simulink model "CyberDog_Motor_FOC_preRefactor_20260807_213408"  (R2025b)
settings: Solver=FixedStepDiscrete  StartTime=0.0  StopTime=0.5  FixedStep=0.0001  RelTol=1e-3
InitFcn:
  | p = fileparts(get_param(bdroot,'FileName')); addpath(fullfile(p,'scripts')); motor_params;
undefined symbols (not defined in the file): Cogging_Lut_Angle, Cogging_Lut_V, CoggingFF_En, Curr_MaxOut, Curr_MinOut, CurrD_Ki, CurrD_Kp, CurrQ_Ki, CurrQ_Kp, DeadComp_En, DeadComp_Lut_I, DeadComp_Lut_V, DiscIntNeverNeededParam, MaxMod, Speed_Ki, Speed_Kp, Speed_Loop_N, Speed_MaxOut, Speed_MinOut, Vbus_nom
settings Model: Creator=Baseline  LastModifiedBy=Baseline

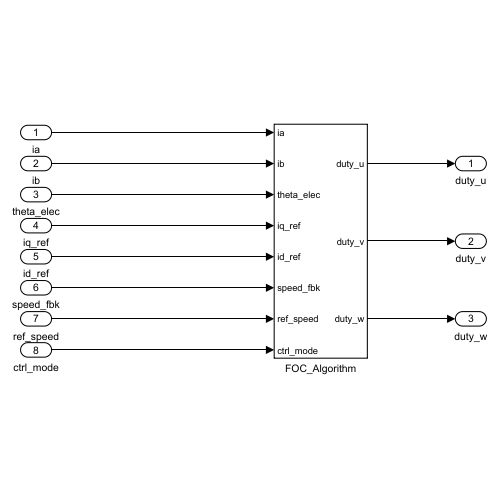
[thumbnail: Simulink's stored preview of the top-level diagram]
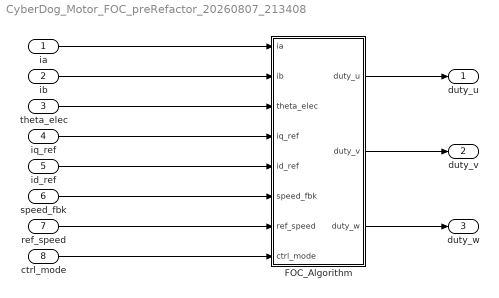
== system CyberDog_Motor_FOC_preRefactor_20260807_213408 ==
  ia : Inport
  ib : Inport  Port=2
  theta_elec : Inport  Port=3
  iq_ref : Inport  Port=4
  id_ref : Inport  Port=5
  speed_fbk : Inport  Port=6
  ref_speed : Inport  Port=7
  ctrl_mode : Inport  Port=8
  FOC_Algorithm : Subsystem
  duty_u : Outport
  duty_v : Outport  Port=2
  duty_w : Outport  Port=3
  wires:
  ctrl_mode/1 -> FOC_Algorithm/8(ctrl_mode)
  ref_speed/1 -> FOC_Algorithm/7(ref_speed)
  speed_fbk/1 -> FOC_Algorithm/6(speed_fbk)
  ia/1 -> FOC_Algorithm/1(ia)
  ib/1 -> FOC_Algorithm/2(ib)
  theta_elec/1 -> FOC_Algorithm/3(theta_elec)
  iq_ref/1 -> FOC_Algorithm/4(iq_ref)
  id_ref/1 -> FOC_Algorithm/5(id_ref)
  FOC_Algorithm/1(duty_u) -> duty_u/1
  FOC_Algorithm/2(duty_v) -> duty_v/1
  FOC_Algorithm/3(duty_w) -> duty_w/1

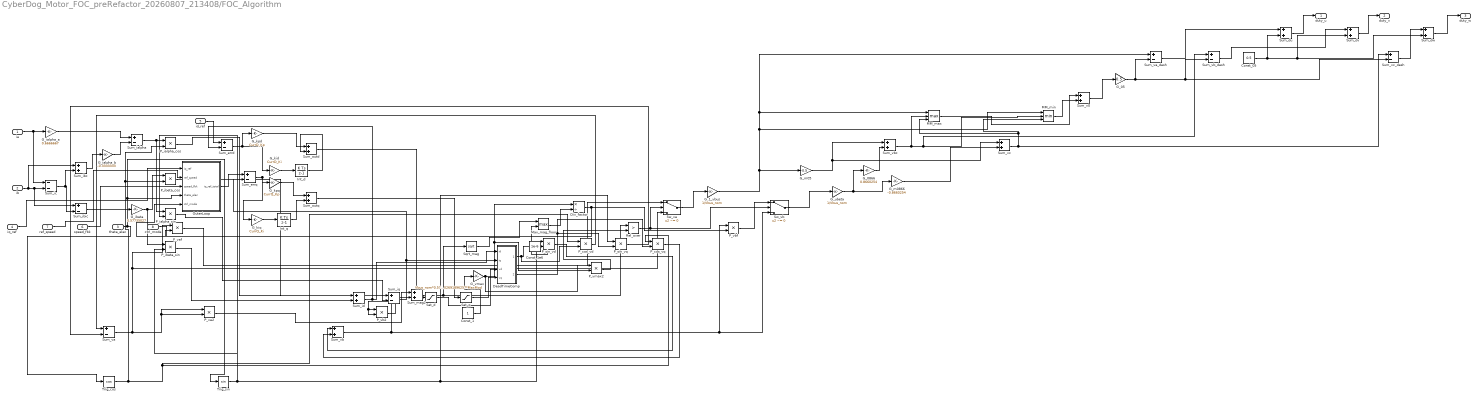
== system CyberDog_Motor_FOC_preRefactor_20260807_213408/FOC_Algorithm ==
  ia : Inport
  ib : Inport  Port=2
  theta_elec : Inport  Port=3
  iq_ref : Inport  Port=4
  id_ref : Inport  Port=5
  speed_fbk : Inport  Port=6
  ref_speed : Inport  Port=7
  ctrl_mode : Inport  Port=8
  Const_05 : Constant  Value=0.5
  Const_1 : Constant
  Const_1e6 : Constant  Value=1e-6
  DeadTimeComp : Subsystem
  Div_factor : Product  Inputs=*/
  G_05 : Gain  Gain=0.5
  G_0866 : Gain  Gain=0.8660254
  G_1_vbus : Gain  Gain=1/Vbus_nom
  G_ialpha_a : Gain  Gain=0.6666667
  G_ialpha_b : Gain  Gain=-0.3333333
  G_ibeta : Gain  Gain=0.57735027
  G_kid : Gain  Gain=CurrD_Ki
  G_kiq : Gain  Gain=CurrQ_Ki
  G_kpd : Gain  Gain=CurrD_Kp
  G_kpq : Gain  Gain=CurrQ_Kp
  G_m05 : Gain  Gain=-0.5
  G_m0866 : Gain  Gain=-0.8660254
  G_ubeta : Gain  Gain=1/Vbus_nom
  G_vmax : Gain  Gain=Vbus_nom*0.5773502691896257*MaxMod
  Int_d : DiscreteIntegrator  SampleTime=-1  LimitOutput=on  UpperSaturationLimit=Curr_MaxOut  LowerSaturationLimit=Curr_MinOut  ICPrevOutput=DiscIntNeverNeededParam  ICPrevScaledInput=DiscIntNeverNeededParam
  Int_q : DiscreteIntegrator  SampleTime=-1  LimitOutput=on  UpperSaturationLimit=Curr_MaxOut  LowerSaturationLimit=Curr_MinOut  ICPrevOutput=DiscIntNeverNeededParam  ICPrevScaledInput=DiscIntNeverNeededParam
  MM_max : MinMax  Function=max  Inputs=3
  MM_min : MinMax  Inputs=3
  Max_mag_floor : MinMax  Function=max  Inputs=2
  OuterLoop : Subsystem
  P_cos_vd : Product  Inputs=**
  P_cos_vq : Product  Inputs=**
  P_ialpha_cos : Product  Inputs=**
  P_ialpha_sin : Product  Inputs=**
  P_ibeta_cos : Product  Inputs=**
  P_ibeta_sin : Product  Inputs=**
  P_sin_vd : Product  Inputs=**
  P_sin_vq : Product  Inputs=**
  P_va2 : Product  Inputs=**
  P_vaf : Product  Inputs=**
  P_vb2 : Product  Inputs=**
  P_vbf : Product  Inputs=**
  P_vmax2 : Product  Inputs=**
  Rel_over : RelationalOperator  Operator=>  OutDataTypeStr=boolean  RndMeth=Simplest  InputSameDT=off
  Sat_d : Saturate  UpperLimit=Curr_MaxOut  LowerLimit=Curr_MinOut
  Sat_q : Saturate  UpperLimit=Curr_MaxOut  LowerLimit=Curr_MinOut
  Sqrt_mag : Sqrt
  Sum_du : Sum
  Sum_dv : Sum
  Sum_dw : Sum
  Sum_errd : Sum  Inputs=+-
  Sum_errq : Sum  Inputs=+-
  Sum_ialpha : Sum  Inputs=+-
  Sum_ibc : Sum
  Sum_ibic : Sum  Inputs=+-
  Sum_ic : Sum  Inputs=--
  Sum_id : Sum
  Sum_iq : Sum  Inputs=+-
  Sum_mag2 : Sum
  Sum_outd : Sum
  Sum_outq : Sum
  Sum_v0 : Sum
  Sum_va : Sum  Inputs=+-
  Sum_va_dash : Sum  Inputs=+-
  Sum_vb : Sum
  Sum_vb_dash : Sum  Inputs=+-
  Sum_vbc : Sum
  Sum_vc : Sum
  Sum_vc_dash : Sum  Inputs=+-
  Sw_va : Switch  Criteria=u2 ~= 0  SaturateOnIntegerOverflow=off  InputSameDT=off
  Sw_vb : Switch  Criteria=u2 ~= 0  SaturateOnIntegerOverflow=off  InputSameDT=off
  Trig_cos : Trigonometry  Operator=cos
  Trig_sin : Trigonometry
  duty_u : Outport
  duty_v : Outport  Port=2
  duty_w : Outport  Port=3
  wires:
  G_kpd/1 -> Sum_outd/1
  id_ref/1 -> Sum_errd/1
  Int_q/1 -> Sum_outq/2
  G_kiq/1 -> Int_q/1
  G_ibeta/1 -> P_ibeta_cos/1, P_ibeta_sin/1
  Sum_ialpha/1 -> P_ialpha_sin/1, P_ialpha_cos/1
  Sum_ibic/1 -> G_ibeta/1
  G_ialpha_b/1 -> Sum_ialpha/2
  G_ialpha_a/1 -> Sum_ialpha/1
  Sum_ibc/1 -> G_ialpha_b/1
  Sum_ic/1 -> Sum_ibic/2, Sum_ibc/2
  ib/1 -> Sum_ibic/1, Sum_ic/2, Sum_ibc/1
  ia/1 -> G_ialpha_a/1, Sum_ic/1
  Sum_dw/1 -> duty_w/1
  Sum_dv/1 -> duty_v/1
  Sum_du/1 -> duty_u/1
  Sum_vc_dash/1 -> Sum_dw/1
  Sum_vb_dash/1 -> Sum_dv/1
  Const_05/1 -> Sum_dw/2, Sum_dv/2, Sum_du/2
  Sum_va_dash/1 -> Sum_du/1
  G_05/1 -> Sum_vc_dash/2, Sum_vb_dash/2, Sum_va_dash/2
  Sum_v0/1 -> G_05/1
  MM_min/1 -> Sum_v0/2
  MM_max/1 -> Sum_v0/1
  Sum_vc/1 -> MM_min/3, MM_max/3, Sum_vc_dash/1
  Sum_vbc/1 -> Sum_vb_dash/1, MM_min/2, MM_max/2
  G_m0866/1 -> Sum_vc/2
  G_0866/1 -> Sum_vbc/2
  G_m05/1 -> Sum_vc/1, Sum_vbc/1
  G_ubeta/1 -> G_m0866/1, G_0866/1
  G_1_vbus/1 -> Sum_va_dash/1, MM_max/1, MM_min/1, G_m05/1
  Sw_vb/1 -> G_ubeta/1
  Sw_va/1 -> G_1_vbus/1
  P_vbf/1 -> Sw_vb/1
  Rel_over/1 -> Sw_vb/2, Sw_va/2
  P_vb2/1 -> Sum_mag2/2
  P_va2/1 -> Sum_mag2/1
  Sum_vb/1 -> Sw_vb/3, P_vbf/1, P_vb2/2, P_vb2/1
  Max_mag_floor/1 -> Div_factor/2
  Sum_mag2/1 -> Rel_over/1, Sqrt_mag/1
  Sqrt_mag/1 -> Max_mag_floor/1
  OuterLoop/1(iq_ref_total) -> Sum_errq/1
  ctrl_mode/1 -> OuterLoop/5(ctrl_mode)
  speed_fbk/1 -> OuterLoop/3(speed_fbk)
  ref_speed/1 -> OuterLoop/2(ref_speed)
  Div_factor/1 -> P_vbf/2, P_vaf/2
  theta_elec/1 -> OuterLoop/4(theta_elec), Trig_sin/1, Trig_cos/1
  Sum_va/1 -> P_va2/1, P_va2/2, P_vaf/1, Sw_va/3
  P_vaf/1 -> Sw_va/1
  iq_ref/1 -> OuterLoop/1(iq_ref)
  Sum_errq/1 -> G_kpq/1, G_kiq/1
  G_kpq/1 -> Sum_outq/1
  Sum_errd/1 -> G_kpd/1, G_kid/1
  G_kid/1 -> Int_d/1
  Int_d/1 -> Sum_outd/2
  DeadTimeComp/2(vq_out) -> P_cos_vq/2, P_sin_vq/2
  DeadTimeComp/1(vd_out) -> P_sin_vd/2, P_cos_vd/2
  Sum_iq/1 -> DeadTimeComp/2(iq), Sum_errq/2
  P_ialpha_sin/1 -> Sum_iq/2
  P_ibeta_cos/1 -> Sum_iq/1
  G_vmax/1 -> P_vmax2/2, Div_factor/1, P_vmax2/1
  Const_1e6/1 -> Max_mag_floor/2
  Sum_outd/1 -> Sat_d/1
  Sum_outq/1 -> Sat_q/1
  Trig_sin/1 -> P_sin_vq/1, P_sin_vd/1, P_ialpha_sin/2, P_ibeta_sin/2
  Trig_cos/1 -> P_cos_vd/1, P_cos_vq/1, P_ibeta_cos/2, P_ialpha_cos/2
  Sat_d/1 -> DeadTimeComp/3(vd)
  Sat_q/1 -> DeadTimeComp/4(vq)
  P_cos_vd/1 -> Sum_va/1
  P_sin_vq/1 -> Sum_va/2
  P_sin_vd/1 -> Sum_vb/1
  P_cos_vq/1 -> Sum_vb/2
  Const_1/1 -> G_vmax/1
  P_vmax2/1 -> Rel_over/2
  P_ialpha_cos/1 -> Sum_id/1
  P_ibeta_sin/1 -> Sum_id/2
  Sum_id/1 -> DeadTimeComp/1(id), Sum_errd/2

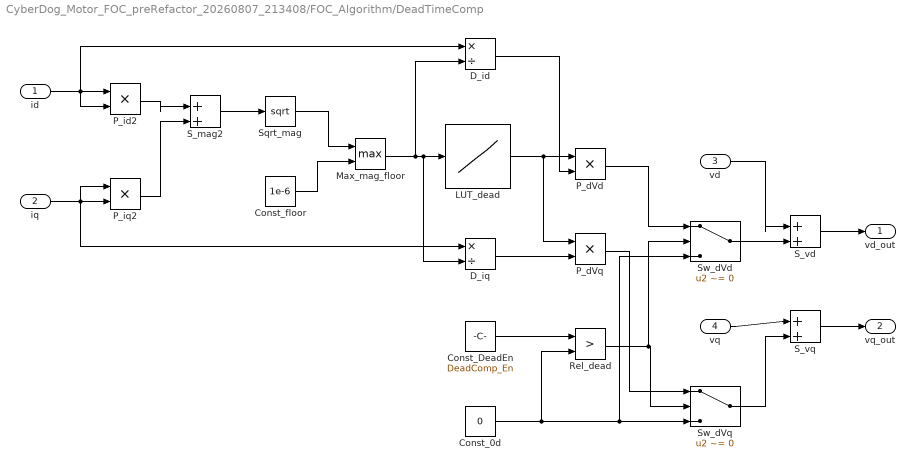
== system CyberDog_Motor_FOC_preRefactor_20260807_213408/FOC_Algorithm/DeadTimeComp ==
  id : Inport
  iq : Inport  Port=2
  vd : Inport  Port=3
  vq : Inport  Port=4
  Const_0d : Constant  Value=0
  Const_DeadEn : Constant  Value=DeadComp_En
  Const_floor : Constant  Value=1e-6
  D_id : Product  Inputs=*/
  D_iq : Product  Inputs=*/
  LUT_dead : Lookup_n-D  NumberOfTableDimensions=1  BreakpointsForDimension1=DeadComp_Lut_I  Table=DeadComp_Lut_V  InternalRulePriority=Speed  RndMeth=Simplest
  Max_mag_floor : MinMax  Function=max  Inputs=2
  P_dVd : Product  Inputs=**
  P_dVq : Product  Inputs=**
  P_id2 : Product  Inputs=**
  P_iq2 : Product  Inputs=**
  Rel_dead : RelationalOperator  Operator=>  OutDataTypeStr=boolean  RndMeth=Simplest  InputSameDT=off
  S_mag2 : Sum  Inputs=|++
  S_vd : Sum  Inputs=|++
  S_vq : Sum  Inputs=|++
  Sqrt_mag : Sqrt
  Sw_dVd : Switch  Criteria=u2 ~= 0  SaturateOnIntegerOverflow=off  InputSameDT=off
  Sw_dVq : Switch  Criteria=u2 ~= 0  SaturateOnIntegerOverflow=off  InputSameDT=off
  vd_out : Outport
  vq_out : Outport  Port=2
  wires:
  S_vq/1 -> vq_out/1
  S_vd/1 -> vd_out/1
  Sw_dVq/1 -> S_vq/2
  vq/1 -> S_vq/1
  Sw_dVd/1 -> S_vd/2
  vd/1 -> S_vd/1
  Const_DeadEn/1 -> Rel_dead/1
  P_dVq/1 -> Sw_dVq/1
  Const_0d/1 -> Sw_dVd/3, Sw_dVq/3, Rel_dead/2
  Rel_dead/1 -> Sw_dVd/2, Sw_dVq/2
  P_dVd/1 -> Sw_dVd/1
  D_iq/1 -> P_dVq/2
  D_id/1 -> P_dVd/2
  LUT_dead/1 -> P_dVd/1, P_dVq/1
  Max_mag_floor/1 -> LUT_dead/1, D_iq/2, D_id/2
  Const_floor/1 -> Max_mag_floor/2
  Sqrt_mag/1 -> Max_mag_floor/1
  S_mag2/1 -> Sqrt_mag/1
  P_iq2/1 -> S_mag2/2
  P_id2/1 -> S_mag2/1
  iq/1 -> D_iq/1, P_iq2/1, P_iq2/2
  id/1 -> P_id2/1, P_id2/2, D_id/1

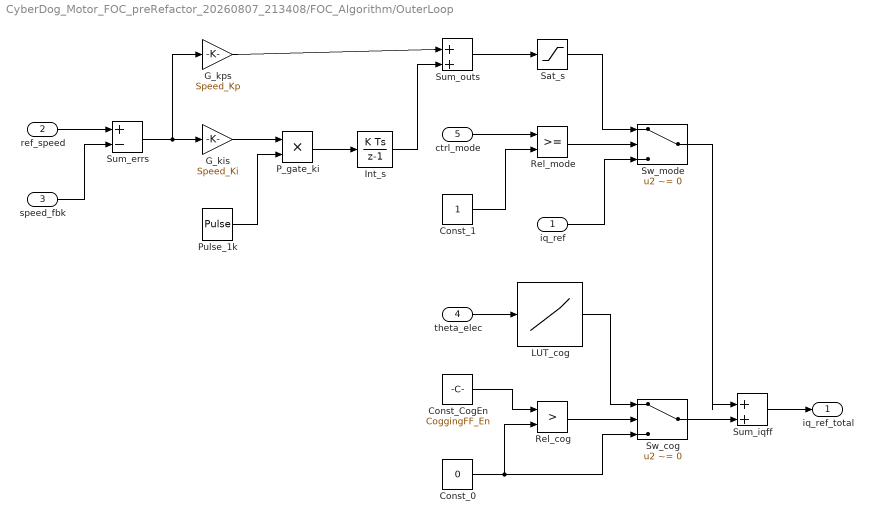
== system CyberDog_Motor_FOC_preRefactor_20260807_213408/FOC_Algorithm/OuterLoop ==
  iq_ref : Inport
  ref_speed : Inport  Port=2
  speed_fbk : Inport  Port=3
  theta_elec : Inport  Port=4
  ctrl_mode : Inport  Port=5
  Const_0 : Constant  Value=0
  Const_1 : Constant
  Const_CogEn : Constant  Value=CoggingFF_En
  G_kis : Gain  Gain=Speed_Ki
  G_kps : Gain  Gain=Speed_Kp
  Int_s : DiscreteIntegrator  SampleTime=-1  LimitOutput=on  UpperSaturationLimit=Speed_MaxOut  LowerSaturationLimit=Speed_MinOut  ICPrevOutput=DiscIntNeverNeededParam  ICPrevScaledInput=DiscIntNeverNeededParam
  LUT_cog : Lookup_n-D  NumberOfTableDimensions=1  BreakpointsForDimension1=Cogging_Lut_Angle  Table=Cogging_Lut_V  InternalRulePriority=Speed  RndMeth=Simplest
  P_gate_ki : Product  Inputs=**
  Pulse_1k : DiscretePulseGenerator  Period=Speed_Loop_N  SampleTime=0.0001
  Rel_cog : RelationalOperator  Operator=>  OutDataTypeStr=boolean  RndMeth=Simplest  InputSameDT=off
  Rel_mode : RelationalOperator  OutDataTypeStr=boolean  RndMeth=Simplest  InputSameDT=off
  Sat_s : Saturate  UpperLimit=Speed_MaxOut  LowerLimit=Speed_MinOut
  Sum_errs : Sum  Inputs=+-
  Sum_iqff : Sum  Inputs=|++
  Sum_outs : Sum  Inputs=|++
  Sw_cog : Switch  Criteria=u2 ~= 0  SaturateOnIntegerOverflow=off  InputSameDT=off
  Sw_mode : Switch  Criteria=u2 ~= 0  SaturateOnIntegerOverflow=off  InputSameDT=off
  iq_ref_total : Outport
  wires:
  Sum_iqff/1 -> iq_ref_total/1
  Sw_cog/1 -> Sum_iqff/2
  Sw_mode/1 -> Sum_iqff/1
  Const_CogEn/1 -> Rel_cog/1
  Const_0/1 -> Sw_cog/3, Rel_cog/2
  Rel_cog/1 -> Sw_cog/2
  LUT_cog/1 -> Sw_cog/1
  theta_elec/1 -> LUT_cog/1
  Const_1/1 -> Rel_mode/2
  ctrl_mode/1 -> Rel_mode/1
  iq_ref/1 -> Sw_mode/3
  Rel_mode/1 -> Sw_mode/2
  Sat_s/1 -> Sw_mode/1
  Sum_outs/1 -> Sat_s/1
  Int_s/1 -> Sum_outs/2
  G_kps/1 -> Sum_outs/1
  P_gate_ki/1 -> Int_s/1
  Pulse_1k/1 -> P_gate_ki/2
  G_kis/1 -> P_gate_ki/1
  Sum_errs/1 -> G_kps/1, G_kis/1
  speed_fbk/1 -> Sum_errs/2
  ref_speed/1 -> Sum_errs/1
